simulink model "Orbit_prop_279C_v2"  (R2018b)
settings: Solver=ode113  StartTime=0.0  StopTime=3600*24*50  FixedStep=25  RelTol=1e-8  AbsTol=1e-10
undefined symbols (not defined in the file or in its folder): DCM, I_vec, mu, mu1, omega, r0, v0, w0
settings Model: Creator=ayotundedemuren  LastModifiedBy=Ethan
settings SolverCC: AutoScaleAbsTol=off

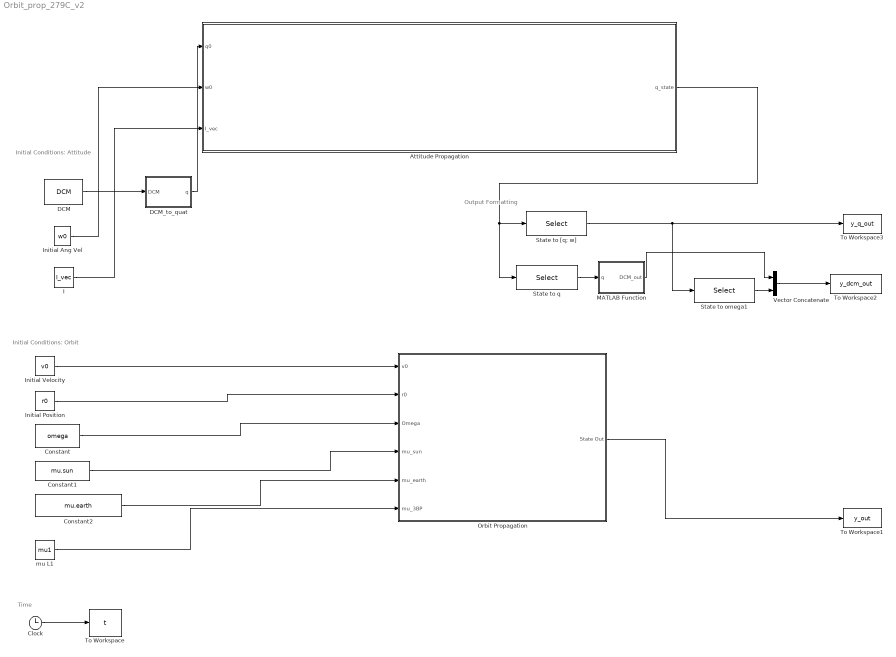
== system Orbit_prop_279C_v2 ==
  note: Output Formatting
  note: Time
  note: Initial Conditions: Orbit
  note: Initial Conditions: Attitude
  Attitude Propagation : Subsystem
  Clock : Clock
      settings: Decimation=100
  Constant : Constant  Value=omega
  Constant1 : Constant  Value=mu.sun
  Constant2 : Constant  Value=mu.earth
  DCM : Constant  Value=DCM
  DCM_to_quat : MATLAB Function  TreatAsAtomicUnit=on
  I : Constant  Value=I_vec
  Initial Ang Vel : Constant  Value=w0
  Initial Position : Constant  Value=r0
  Initial Velocity : Constant  Value=v0
  MATLAB Function : MATLAB Function  TreatAsAtomicUnit=on
  Orbit Propagation : Subsystem
  State to [q; w] : Selector  InputPortWidth=10  IndexOptions=Starting index (dialog)  Indices=[1]  OutputSizes=7
  State to omega1 : Selector  InputPortWidth=7  IndexOptions=Starting index (dialog)  Indices=5  OutputSizes=3
  State to q : Selector  InputPortWidth=10  IndexOptions=Starting index (dialog)  Indices=[1]  OutputSizes=4
  To Workspace : ToWorkspace  VariableName=t  SampleTime=-1
      settings: Save2DSignal=2-D array (concatenate along first dimension)
  To Workspace1 : ToWorkspace  VariableName=y_out  SampleTime=-1
  To Workspace2 : ToWorkspace  VariableName=y_dcm_out  SampleTime=-1
      settings: Save2DSignal=2-D array (concatenate along first dimension)
  To Workspace3 : ToWorkspace  VariableName=y_q_out  SampleTime=-1
  Vector Concatenate : Concatenate
  mu L1 : Constant  Value=mu1
  wires:
  Clock/1 -> To Workspace/1
  DCM/1 -> DCM_to_quat/1(DCM)
  Initial Velocity/1 -> Orbit Propagation/1(v0)
  Initial Position/1 -> Orbit Propagation/2(r0)
  Constant/1 -> Orbit Propagation/3(Omega)
  Constant1/1 -> Orbit Propagation/4(mu_sun)
  Constant2/1 -> Orbit Propagation/5(mu_earth)
  mu L1/1 -> Orbit Propagation/6(mu_3BP)
  Orbit Propagation/1(State Out) -> To Workspace1/1
  State to [q; w]/1 -> State to omega1/1, To Workspace3/1
  State to q/1 -> MATLAB Function/1(q)
  MATLAB Function/1(DCM_out) -> Vector Concatenate/1
  State to omega1/1 -> Vector Concatenate/2
  Vector Concatenate/1 -> To Workspace2/1
  Attitude Propagation/1(q_state) -> State to q/1, State to [q; w]/1
  DCM_to_quat/1(q) -> Attitude Propagation/1(q0)
  Initial Ang Vel/1 -> Attitude Propagation/2(w0)
  I/1 -> Attitude Propagation/3(I_vec)

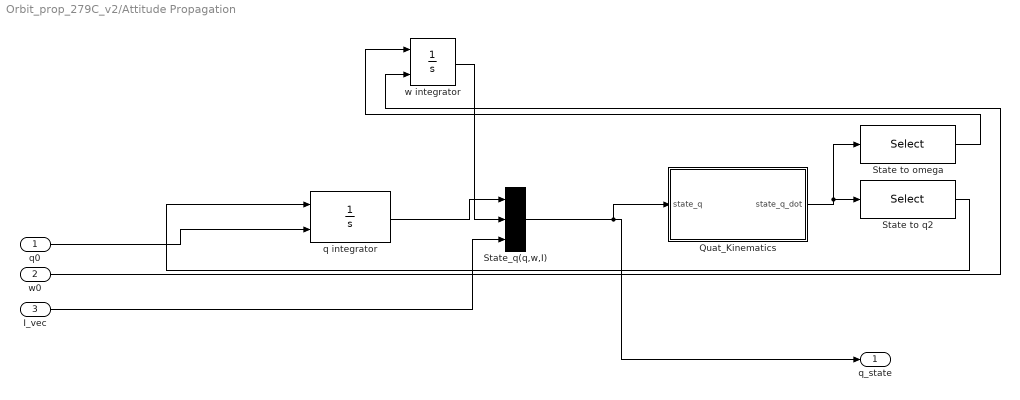
== system Orbit_prop_279C_v2/Attitude Propagation ==
  q0 : Inport
  w0 : Inport  Port=2
  I_vec : Inport  Port=3
  Quat_Kinematics : MATLAB Function  TreatAsAtomicUnit=on
  State to omega : Selector  InputPortWidth=10  IndexOptions=Starting index (dialog)  Indices=5  OutputSizes=3
  State to q2 : Selector  InputPortWidth=10  IndexOptions=Starting index (dialog)  Indices=[1]  OutputSizes=4
  State_q(q,w,I) : Concatenate  NumInputs=3
  q integrator : Integrator  InitialConditionSource=external
  w integrator : Integrator  InitialConditionSource=external
  q_state : Outport
  wires:
  State_q(q,w,I)/1 -> q_state/1, Quat_Kinematics/1(state_q)
  w integrator/1 -> State_q(q,w,I)/2
  q integrator/1 -> State_q(q,w,I)/1
  State to omega/1 -> w integrator/1
  Quat_Kinematics/1(state_q_dot) -> State to omega/1, State to q2/1
  State to q2/1 -> q integrator/1
  w0/1 -> w integrator/2
  q0/1 -> q integrator/2
  I_vec/1 -> State_q(q,w,I)/3

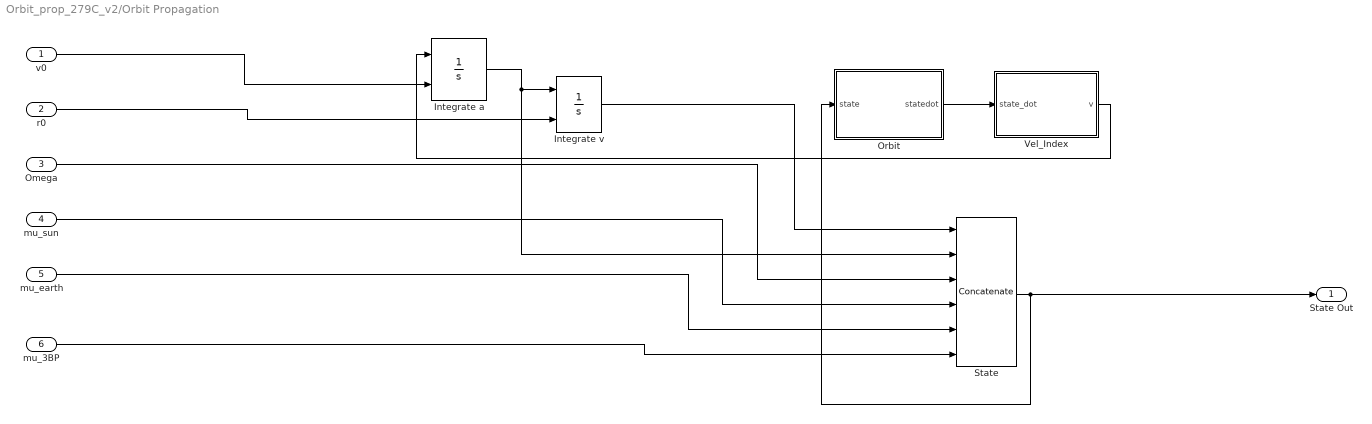
== system Orbit_prop_279C_v2/Orbit Propagation ==
  v0 : Inport
  r0 : Inport  Port=2
  Omega : Inport  Port=3
  mu_sun : Inport  Port=4
  mu_earth : Inport  Port=5
  mu_3BP : Inport  Port=6
  Integrate a : Integrator  InitialConditionSource=external  AbsoluteTolerance=1e-6
  Integrate v : Integrator  InitialConditionSource=external  AbsoluteTolerance=1e-6
  Orbit : MATLAB Function  TreatAsAtomicUnit=on
  "State " : Concatenate  NumInputs=6
  Vel_Index : MATLAB Function  TreatAsAtomicUnit=on
  State Out : Outport
  wires:
  r0/1 -> Integrate v/2
  Integrate a/1 -> Integrate v/1, "State "/2
  Integrate v/1 -> "State "/1
  "State "/1 -> Orbit/1(state), State Out/1
  Vel_Index/1(v) -> Integrate a/1
  Orbit/1(statedot) -> Vel_Index/1(state_dot)
  v0/1 -> Integrate a/2
  mu_3BP/1 -> "State "/6
  Omega/1 -> "State "/3
  mu_sun/1 -> "State "/4
  mu_earth/1 -> "State "/5

== matlab function Orbit_prop_279C_v2/Orbit Propagation/Vel_Index ==
  data: state_dot input; v output
function v = fcn(state_dot)

v = state_dot(4:6);

end

== matlab function Orbit_prop_279C_v2/Orbit Propagation/Orbit ==
  data: state input; statedot output
function statedot = fcn(state)

dis_sun = 149599650;

statedot = zeros(length(state),1);
x = state(1);
y = state(2);
z = state(3);
xdot = state(4);
ydot = state(5);
zdot = state(6);

w = state(7);
mu1 = state(8);
mu2 = state(9);
mu_sys = state(10);

Rx1 = - mu_sys*dis_sun;
Rx2 = (1-mu_sys)*dis_sun;

R1 = sqrt((x - Rx1)^2 + y^2 + z^2);
R2 = sqrt((x - Rx2)^2 + y^2 + z^2);

statedot(1) = xdot;
statedot(2) = ydot;
statedot(3) = zdot;

statedot(4) = x*w^2 + 2*ydot*w + mu1 * (Rx1 - x)/R1^3 + mu2 * (Rx2 - x)/R2^3;
statedot(5) = y*w^2 - 2*xdot*w - mu1 * (y)/R1^3 - mu2 * (y)/R2^3; 
statedot(6) = - mu1 * (z)/R1^3 - mu2 * (z)/R2^3;
end

== matlab function Orbit_prop_279C_v2/Attitude Propagation/Quat_Kinematics ==
  data: state_q input; state_q_dot output
function state_q_dot  = quat_kin(state_q)
% state = [q1 q2 q3 q4 w1 w2 w3 I1 I2 I3]

state_q_dot = zeros(length(state_q),1);
wx = state_q(5);
wy = state_q(6);
wz = state_q(7);
%% Kinematic Equations
Omega = [0 wz -wy wx; -wz 0 wx wy; wy -wx 0 wz; -wx -wy -wz 0];
err = 1 - norm(state_q(1:4));
state_q_dot(1:4) = 1/2 * Omega * state_q(1:4) + 0.05 * err * state_q(1:4);

%% Euler Equations
state_q_dot(5:end) = euler_eq(state_q(5:end));
% state_q_dot(5) = -wy*wz * (state_q(10) - state_q(9))/state_q(8);
% state_q_dot(6) = -wx*wz * (state_q(8) - state_q(10))/state_q(9);
% state_q_dot(7) = -wx*wy * (state_q(9) - state_q(8))/state_q(10);

end

== matlab function Orbit_prop_279C_v2/DCM_to_quat ==
  data: DCM input; q output
function q  = DCM_to_quat(DCM)
B4 = 1/4 * (1 + trace(DCM));
B1 = 1/4 * (1 + 2*DCM(1,1) - trace(DCM));
B2 = 1/4 * (1 + 2*DCM(2,2) - trace(DCM));
B3 = 1/4 * (1 + 2*DCM(3,3) - trace(DCM));
B = [B1 B2 B3 B4];
[M, I] = max(B);
q = zeros(4,1);
q(4) = sqrt(B(I));
if I == 4
    q(1) = (DCM(2,3) - DCM(3,2)) / 4 / q(4);
    q(2) = (DCM(3,1) - DCM(1,3)) / 4 / q(4);
    q(3) = (DCM(1,2) - DCM(2,1)) / 4 / q(4);
elseif I == 3
    q(2) = (DCM(2,3) + DCM(3,2)) / 4 / q(4);
    q(1) = (DCM(3,1) + DCM(1,3)) / 4 / q(4);
    q(3) = (DCM(1,2) - DCM(2,1)) / 4 / q(4);
elseif I == 2
    q(2) = (DCM(2,3) + DCM(3,2)) / 4 / q(4);
    q(3) = (DCM(3,1) - DCM(1,3)) / 4 / q(4);
    q(1) = (DCM(1,2) + DCM(2,1)) / 4 / q(4);
elseif I == 1
    q(3) = (DCM(2,3) - DCM(3,2)) / 4 / q(4);
    q(2) = (DCM(3,1) + DCM(1,3)) / 4 / q(4);
    q(1) = (DCM(1,2) + DCM(2,1)) / 4 / q(4);
end
q = q/norm(q);
end

== matlab function Orbit_prop_279C_v2/MATLAB Function ==
  data: q input; DCM_out output
function DCM_out  = quat_to_DCM(q)

DCM = zeros(3, 3);
DCM(:, :) = ((q(4)^2 - norm(q(1:3))^2)*eye(3) ...
    + 2 * q(1:3) * q(1:3)'...
    - 2 * q(4) * ...
    [0, -q(3), q(2); q(3), 0, -q(1); ...
    -q(2), q(1), 0]);

DCM_out = DCM(:)';
end
